simulink model "ExciterFlowCurrent_NoLoadSwitch"  (R2015a)
settings: Solver=ode45  StartTime=0.0  StopTime=1  RelTol=1e-3
undefined symbols (not defined in the file or in its folder): D11, Delta
libraries: powerlib x9
settings Model: Creator=baishuhua  LastModifiedBy=baishuhua
settings DebuggingCC: AlgebraicLoopMsg=none

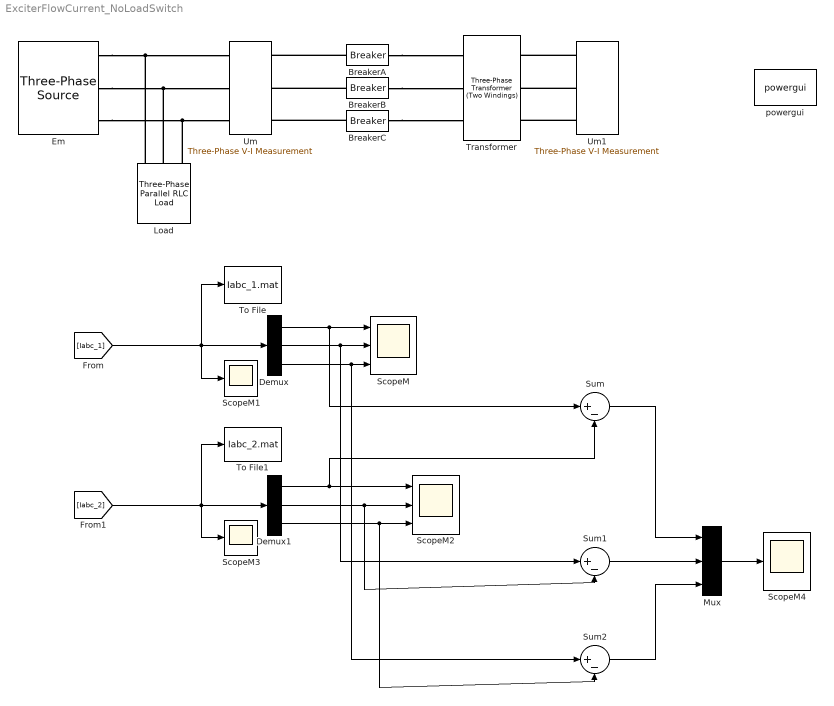
== system ExciterFlowCurrent_NoLoadSwitch ==
  BreakerA : powerlib/Elements/Breaker  InitialState=0  SwitchingTimes=[0.1 1]  External=off  BreakerResistance=0.01  SnubberResistance=1e6  SnubberCapacitance=inf  Measurements=None  MoreParameters=on  NoBreakLoop=off
  BreakerB : powerlib/Elements/Breaker  InitialState=0  SwitchingTimes=[0.2 1]  External=off  BreakerResistance=0.01  SnubberResistance=1e6  SnubberCapacitance=inf  Measurements=None  MoreParameters=on  NoBreakLoop=off
  BreakerC : powerlib/Elements/Breaker  InitialState=0  SwitchingTimes=[0.3 1]  External=off  BreakerResistance=0.01  SnubberResistance=1e6  SnubberCapacitance=inf  Measurements=None  MoreParameters=on  NoBreakLoop=off
  Demux : Demux  Outputs=3
  Demux1 : Demux  Outputs=3
  Em : powerlib/Electrical Sources/Three-Phase Source  Voltage=35e3  PhaseAngle=180  Frequency=50  InternalConnection=Yg  SpecifyImpedance=off  Resistance=0.8929  Inductance=16.58e-3  ShortCircuitLevel=100e6  BaseVoltage=35e3  XRratio=7  BusType=swing  Pref=0  Qref=0  Qmin=-inf  Qmax=inf
  Load : powerlib/Elements/Three-Phase Parallel RLC Load  LConnTagsString=A|B|C  Configuration=Y (grounded)  NominalVoltage=35e3  NominalFrequency=50  ActivePower=30e6  InductivePower=0  CapacitivePower=1e6  Measurements=None  LoadType=constant PQ
  Mux : Mux  Inputs=3
  ScopeM : Scope  NumInputPorts=3
      settings: ShowLegends=on  TimeRange=1  YMin=-500~-4000~-1750  YMax=4000~500~250  SampleInput=on
  ScopeM1 : Scope
      settings: ShowLegends=on  TimeRange=1  YMin=-500  YMax=4000  SampleInput=on
  ScopeM2 : Scope  NumInputPorts=3
      settings: ShowLegends=on  TimeRange=1  YMin=-500~-4000~-1750  YMax=4000~500~250  SaveName=ScopeData2  SampleInput=on
  ScopeM3 : Scope
      settings: ShowLegends=on  TimeRange=1  YMin=-500  YMax=4000  SaveName=ScopeData3  SampleInput=on
  ScopeM4 : Scope
      settings: ShowLegends=on  TimeRange=1  YMin=-500  YMax=4000  SaveName=ScopeData4  SampleInput=on
  Sum : Sum  Inputs=|+-
  Sum1 : Sum  Inputs=|+-
  Sum2 : Sum  Inputs=|+-
  To File : ToFile  Filename=Iabc_1.mat  MatrixName=Iabc_1  SaveFormat=Timeseries
  To File1 : ToFile  Filename=Iabc_2.mat  MatrixName=Iabc_2  SaveFormat=Timeseries
  Transformer : powerlib/Elements/Three-Phase Transformer (Two Windings)  Winding1Connection=Delta (D11)  Winding2Connection=Delta (D11)  CoreType=Three single-phase transformers  SetSaturation=on  Hysteresis=off  DataFile='hysteresis'  SetInitialFlux=on  Measurements=None  UNITS=pu  NominalPower=[300e6 50]  Winding1=[ 35e3 , 0.002 , 0.08 ]  Winding2=[ 220e3 , 0.002 , 0.08 ]  Rm=500  Lm=500  L0=0.5  Saturation=[ 0,0 ; 0.0024,1.2 ; 1.0,1.52 ]  InitialFluxes=[0.5 0 0]  MoreParameters=off  BreakLoop=off  DataType=off  TransfoNumber=1
  Um : powerlib/Measurements/Three-Phase V-I Measurement  VoltageMeasurement=no  SetLabelV=on  LabelV=Vabc_M  Vpu=off  VpuLL=off  CurrentMeasurement=yes  SetLabelI=on  LabelI=Iabc_1  Ipu=on  Pbase=100e6  Vbase=35e3  OutputType=Complex  PhasorSimulation=off  PSBequivalent=0
  Um1 : powerlib/Measurements/Three-Phase V-I Measurement  VoltageMeasurement=no  SetLabelV=on  LabelV=Vabc_M  Vpu=off  VpuLL=off  CurrentMeasurement=yes  SetLabelI=on  LabelI=Iabc_2  Ipu=on  Pbase=100e6  Vbase=220e3  OutputType=Complex  PhasorSimulation=off  PSBequivalent=0
  powergui : powerlib/powergui  Priority=1  SimulationMode=Discrete  SolverType=Tustin/Backward Euler (TBE)  SampleTime=1e-4  frequency=60  SPID=off  DisableSnubberDevices=off  DisableRonSwitches=off  DisableVfSwitches=off  SwTol=0  DisplayEquations=off  Interpol=off  methode=off  Ts=100  FunctionMessages=off  echomessages=off  HookPort=off  EnableUseOfTLC=off  x0status=blocks  frequencyindice=50  Pbase=100e6  ErrMax=1e-4  Iterations=50  UnitsV=kV  UnitsW=MW  buscounter=0  RestoreLinks=warning  ResistiveCurrentMeasurement=off  Frange=[0:2:500]  Ylog=off  Xlog=on  ShowGrid=off  save=off  variable=ZData  structure=0  ZoomFFT=off  StartTime=0.0  cycles=1  DisplayStyle=1  fundamental=60  FreqAxis=off  MaxFrequency=1000  frequencyindicesteady=1  RmsSteady=1  display=off
  wires:
  [Iabc_1] -> ScopeM1/1, To File/1, Demux/1
  Demux/1 -> Sum/1, ScopeM/1
  Demux/2 -> Sum1/1, ScopeM/2
  Demux/3 -> Sum2/1, ScopeM/3
  Demux1/1 -> ScopeM2/1, Sum/2
  Demux1/2 -> Sum1/2, ScopeM2/2
  Demux1/3 -> Sum2/2, ScopeM2/3
  Sum/1 -> Mux/1
  Sum1/1 -> Mux/2
  Sum2/1 -> Mux/3
  Mux/1 -> ScopeM4/1
  [Iabc_2] -> ScopeM3/1, To File1/1, Demux1/1
  connections:
  Em/RConn1 -- Um/LConn1 -- Load/LConn1
  Em/RConn2 -- Um/LConn2 -- Load/LConn2
  Em/RConn3 -- Um/LConn3 -- Load/LConn3
  BreakerA/LConn1 -- Um/RConn1
  BreakerA/RConn1 -- Transformer/LConn1
  BreakerB/RConn1 -- Transformer/LConn2
  BreakerC/RConn1 -- Transformer/LConn3
  BreakerC/LConn1 -- Um/RConn3
  BreakerB/LConn1 -- Um/RConn2
  Um1/LConn1 -- Transformer/RConn1
  Um1/LConn2 -- Transformer/RConn2
  Um1/LConn3 -- Transformer/RConn3
